simulink model "single_camera_xy_tracking_5dof"  (R2025b)
settings: Solver=FixedStepDiscrete  StartTime=0  StopTime=T_end  FixedStep=Ts  RelTol=1e-3
InitFcn:
  | % 获取顶层模型所在文件夹
  | root_model_file = get_param(bdroot,'FileName');
  | root_folder = fileparts(root_model_file);
  | % 定位config目录：模型目录上跳一层 → simulink → config
  | func_folder = fullfile(root_folder,'..','config');
  | addpath(func_folder);
  | % 拼接初始化脚本完整路径
  | init_script = fullfile(func_folder,'init_single_camera_xy_tracking_5dof.m');
  | run(init_script);
values from neighbouring files (symbols this model uses):
  Kpx = parameters(3)    [build_single_camera_joint_velocity_direct.m]    (also in build_single_camera_joint_velocity_direct1.m)
  Kpy = parameters(4);",  "k_ff=parameters(5)    [build_single_camera_joint_velocity_direct.m]    (also in build_single_camera_joint_velocity_direct1.m)
  Z_hat = parameters(2)    [build_single_camera_joint_velocity_direct.m]    (also in build_single_camera_joint_velocity_direct1.m)
undefined symbols (not defined in the file or in its folder): a_xy_max, adapt_max, camera_velocity_feedback_timeout_sec, controller_enable, cx, cy, data, data_SL_Info, ekf_gate_threshold, ekf_reset_timeout_sec, enable_adaptation, enable_ekf_feedforward, enable_proportional, fx, fy, gamma_adapt, joint_state_timeout_sec, k_ff, P0, Q_ekf, R_ekf, sigma_adapt, target_timeout_sec, Ts, v_xy_max
libraries: ros2lib x4, robotmaniplib x2
Description:
  | 5-DOF camera EKF/controller: vx, vy, wx, wy, wz enabled; vz=0.
settings Model: Creator=ASUS  LastModifiedBy=harry
settings DataIOCC: SignalLogging=off

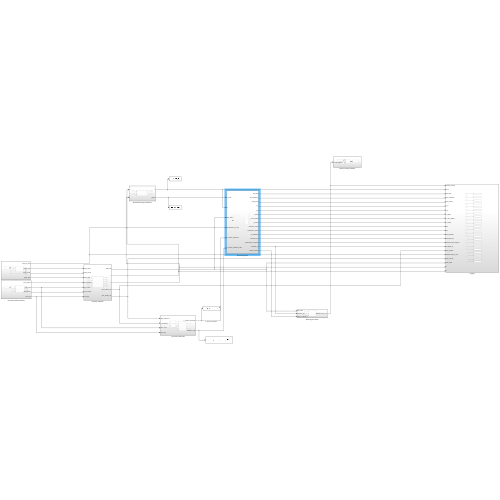
[thumbnail: Simulink's stored preview of the top-level diagram]
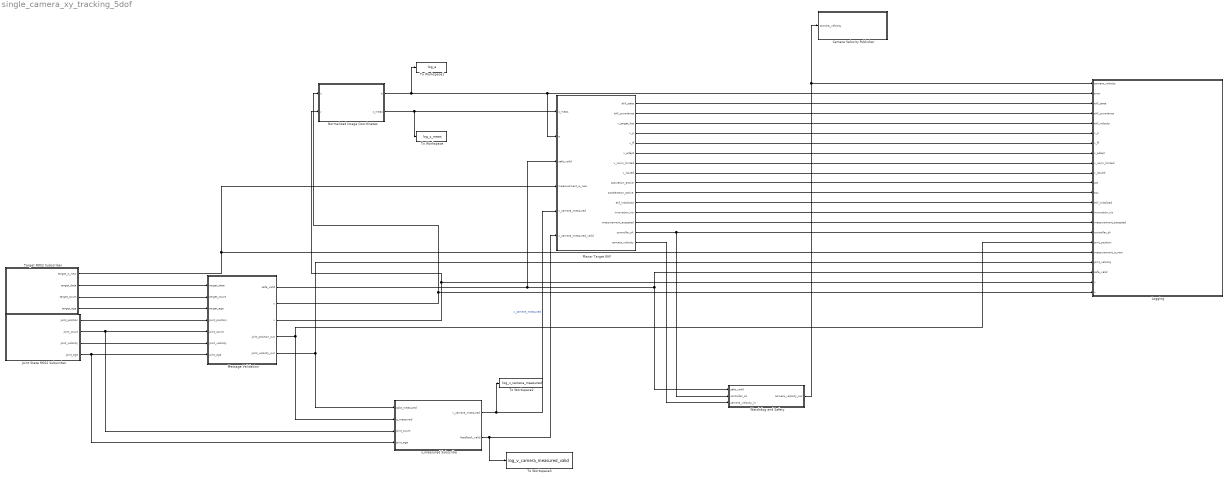
== system single_camera_xy_tracking_5dof ==
  Camera Velocity Publisher : Subsystem
  Joint State ROS2 Subscriber : Subsystem
  Logging : Subsystem
  Message Validation : Subsystem
  Normalized Image Coordinates : Subsystem
  Planar Target EKF : Subsystem
  Target ROS2 Subscriber : Subsystem
  To Workspace : ToWorkspace  VariableName=log_z_meas  SaveFormat=Timeseries  SampleTime=-1
  To Workspace1 : ToWorkspace  VariableName=log_e  SaveFormat=Timeseries  SampleTime=-1
  To Workspace2 : ToWorkspace  VariableName=log_v_camera_measured  SaveFormat=Timeseries  SampleTime=-1
  To Workspace3 : ToWorkspace  VariableName=log_v_camera_measured_valid  SaveFormat=Timeseries  SampleTime=-1
  Watchdog and Safety : Subsystem
  v_measured Subscribe : Subsystem
  wires:
  Target ROS2 Subscriber/4(target_age) -> Message Validation/3(target_age)
  Target ROS2 Subscriber/2(target_data) -> Message Validation/1(target_data)
  Target ROS2 Subscriber/3(target_count) -> Message Validation/2(target_count)
  Planar Target EKF/3(v_target_hat) -> Logging/5(ekf_velocity)
  Message Validation/2(u) -> Normalized Image Coordinates/1(u), Logging/22(u)
  Planar Target EKF/14(controller_ok) -> Watchdog and Safety/2(controller_ok), Logging/16(controller_ok)
  Planar Target EKF/6(v_adapt) -> Logging/8(v_adapt)
  Joint State ROS2 Subscriber/4(joint_age) -> v_measured Subscribe/4(joint_age), Message Validation/7(joint_age)
  Joint State ROS2 Subscriber/2(joint_count) -> v_measured Subscribe/3(joint_count), Message Validation/5(joint_count)
  Joint State ROS2 Subscriber/1(joint_position) -> Message Validation/4(joint_position)
  Joint State ROS2 Subscriber/3(joint_velocity) -> Message Validation/6(joint_velocity)
  Message Validation/1(safe_valid) -> Logging/20(safe_valid), Watchdog and Safety/1(safe_valid), Planar Target EKF/3(safe_valid)
  Message Validation/3(v) -> Normalized Image Coordinates/2(v), Logging/21(v)
  Message Validation/4(joint_position_out) -> v_measured Subscribe/2(q_measured), Logging/17(joint_position)
  Message Validation/5(joint_velocity_out) -> v_measured Subscribe/1(qdot_measured), Logging/19(joint_velocity)
  Normalized Image Coordinates/1(e) -> To Workspace1/1, Logging/2(error), Planar Target EKF/2(e)
  Normalized Image Coordinates/2(z_meas) -> To Workspace/1, Planar Target EKF/1(z_meas)
  Planar Target EKF/1(ekf_state) -> Logging/3(ekf_state)
  Planar Target EKF/2(ekf_covariance) -> Logging/4(ekf_covariance)
  Planar Target EKF/13(measurement_accepted) -> Logging/15(measurement_accepted)
  Planar Target EKF/9(saturation_active) -> Logging/11(sat)
  Planar Target EKF/10(acceleration_active) -> Logging/12(acc)
  Planar Target EKF/11(ekf_initialized) -> Logging/13(ekf_initialized)
  Planar Target EKF/12(innovation_nis) -> Logging/14(innovation_nis)
  Planar Target EKF/4(v_p) -> Logging/6(v_p)
  Planar Target EKF/5(v_ff) -> Logging/7(v_ff)
  Planar Target EKF/8(v_issued) -> Logging/10(v_issued)
  Planar Target EKF/15(camera_velocity) -> Watchdog and Safety/3(camera_velocity_in)
  Watchdog and Safety/1(camera_velocity_out) -> Camera Velocity Publisher/1(camera_velocity), Logging/1(camera_velocity)
  Target ROS2 Subscriber/1(target_is_new) -> Planar Target EKF/4(measurement_is_new), Logging/18(measurement_is_new)
  v_measured Subscribe/1(v_camera_measured) -> To Workspace2/1, Planar Target EKF/5(v_camera_measured)  "v_camera_measured"
  v_measured Subscribe/2(feedback_valid) -> To Workspace3/1, Planar Target EKF/6(v_camera_measured_valid)
  Planar Target EKF/7(v_norm_limited) -> Logging/9(v_norm_limited)

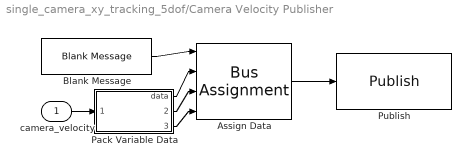
== system single_camera_xy_tracking_5dof/Camera Velocity Publisher ==
  camera_velocity : Inport
  Assign Data : BusAssignment  AssignedSignals=data,data_SL_Info.CurrentLength,data_SL_Info.ReceivedLength
  Blank Message : ros2lib/Blank Message  messageClass=Message  entityType=std_msgs/Float64MultiArray  messageType=std_msgs/Float64MultiArray  SampleTime=Ts
  Pack Variable Data : MATLAB Function  TreatAsAtomicUnit=on
  Publish : ros2lib/Publish  topicSource=Select from ROS network  topic=/simulink/camera_velocity  messageType=std_msgs/Float64MultiArray  QOSHistory=Keep last  QOSDepth=1  QOSReliability=Reliable  QOSDurability=Volatile  QOSDeadline=Inf  QOSLifespan=Inf  QOSLiveliness=Automatic  QOSLeaseDuration=Inf  QOSAvoidROSNamespaceConventions=off
  wires:
  Blank Message/1 -> Assign Data/1
  Assign Data/1 -> Publish/1
  camera_velocity/1 -> Pack Variable Data/1(camera_velocity)
  Pack Variable Data/1(data) -> Assign Data/2
  Pack Variable Data/2(current_length) -> Assign Data/3
  Pack Variable Data/3(received_length) -> Assign Data/4

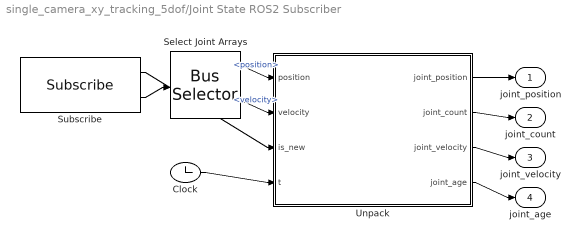
== system single_camera_xy_tracking_5dof/Joint State ROS2 Subscriber ==
  Clock : Clock
  Select Joint Arrays : BusSelector  OutputSignals=position,velocity
  Subscribe : ros2lib/Subscribe  topicSource=Select from ROS network  topic=/franka/joint_states  messageType=sensor_msgs/JointState  sampleTime=Ts  QOSHistory=Keep last  QOSDepth=1  QOSReliability=Best effort  QOSDurability=Volatile  QOSDeadline=Inf  QOSLifespan=Inf  QOSLiveliness=Automatic  QOSLeaseDuration=Inf  QOSAvoidROSNamespaceConventions=off
  Unpack : MATLAB Function  TreatAsAtomicUnit=on
  joint_position : Outport
  joint_count : Outport  Port=2
  joint_velocity : Outport  Port=3
  joint_age : Outport  Port=4
  wires:
  Unpack/1(joint_position) -> joint_position/1
  Unpack/2(joint_count) -> joint_count/1
  Unpack/3(joint_velocity) -> joint_velocity/1
  Unpack/4(joint_age) -> joint_age/1
  Select Joint Arrays/1 -> Unpack/1(position)  "<position>"
  Select Joint Arrays/2 -> Unpack/2(velocity)  "<velocity>"
  Clock/1 -> Unpack/4(t)
  Subscribe/2 -> Select Joint Arrays/1
  Subscribe/1 -> Unpack/3(is_new)

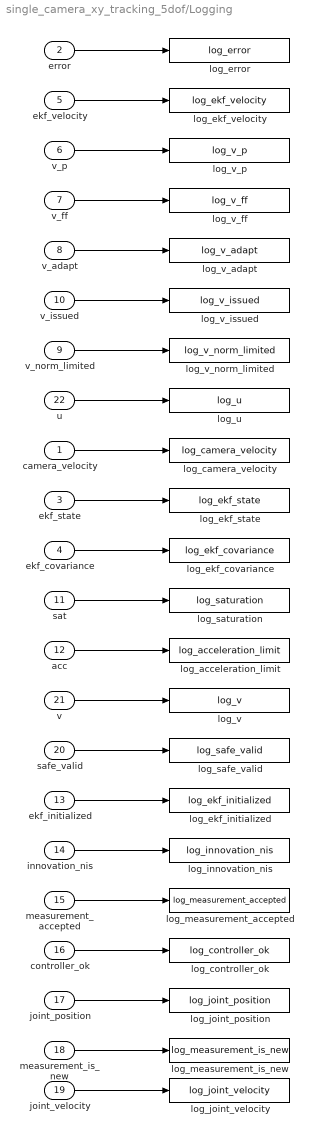
== system single_camera_xy_tracking_5dof/Logging ==
  camera_velocity : Inport
  error : Inport  Port=2
  ekf_state : Inport  Port=3
  ekf_covariance : Inport  Port=4
  ekf_velocity : Inport  Port=5
  v_p : Inport  Port=6
  v_ff : Inport  Port=7
  v_adapt : Inport  Port=8
  v_norm_limited : Inport  Port=9
  v_issued : Inport  Port=10
  sat : Inport  Port=11
  acc : Inport  Port=12
  ekf_initialized : Inport  Port=13
  innovation_nis : Inport  Port=14
  measurement_accepted : Inport  Port=15
  controller_ok : Inport  Port=16
  joint_position : Inport  Port=17
  measurement_is_new : Inport  Port=18
  joint_velocity : Inport  Port=19
  safe_valid : Inport  Port=20
  v : Inport  Port=21
  u : Inport  Port=22
  log_acceleration_limit : ToWorkspace  VariableName=log_acceleration_limit  SaveFormat=Structure With Time  SampleTime=-1
  log_camera_velocity : ToWorkspace  VariableName=log_camera_velocity  SaveFormat=Structure With Time  SampleTime=-1
  log_controller_ok : ToWorkspace  VariableName=log_controller_ok  SaveFormat=Structure With Time  SampleTime=-1
  log_ekf_covariance : ToWorkspace  VariableName=log_ekf_covariance  SaveFormat=Structure With Time  SampleTime=-1
  log_ekf_initialized : ToWorkspace  VariableName=log_ekf_initialized  SaveFormat=Structure With Time  SampleTime=-1
  log_ekf_state : ToWorkspace  VariableName=log_ekf_state  SaveFormat=Structure With Time  SampleTime=-1
  log_ekf_velocity : ToWorkspace  VariableName=log_ekf_velocity  SaveFormat=Structure With Time  SampleTime=-1
  log_error : ToWorkspace  VariableName=log_error  SaveFormat=Structure With Time  SampleTime=-1
  log_innovation_nis : ToWorkspace  VariableName=log_innovation_nis  SaveFormat=Structure With Time  SampleTime=-1
  log_joint_position : ToWorkspace  VariableName=log_joint_position  SaveFormat=Structure With Time  SampleTime=-1
  log_joint_velocity : ToWorkspace  VariableName=log_joint_velocity  SaveFormat=Structure With Time  SampleTime=-1
  log_measurement_accepted : ToWorkspace  VariableName=log_measurement_accepted  SaveFormat=Structure With Time  SampleTime=-1
  log_measurement_is_new : ToWorkspace  VariableName=log_measurement_is_new  SaveFormat=Structure With Time  SampleTime=-1
  log_safe_valid : ToWorkspace  VariableName=log_safe_valid  SaveFormat=Structure With Time  SampleTime=-1
  log_saturation : ToWorkspace  VariableName=log_saturation  SaveFormat=Structure With Time  SampleTime=-1
  log_u : ToWorkspace  VariableName=log_u  SaveFormat=Structure With Time  SampleTime=-1
  log_v : ToWorkspace  VariableName=log_v  SaveFormat=Structure With Time  SampleTime=-1
  log_v_adapt : ToWorkspace  VariableName=log_v_adapt  SaveFormat=Structure With Time  SampleTime=-1
  log_v_ff : ToWorkspace  VariableName=log_v_ff  SaveFormat=Structure With Time  SampleTime=-1
  log_v_issued : ToWorkspace  VariableName=log_v_issued  SaveFormat=Structure With Time  SampleTime=-1
  log_v_norm_limited : ToWorkspace  VariableName=log_v_norm_limited  SaveFormat=Structure With Time  SampleTime=-1
  log_v_p : ToWorkspace  VariableName=log_v_p  SaveFormat=Structure With Time  SampleTime=-1
  wires:
  error/1 -> log_error/1
  ekf_velocity/1 -> log_ekf_velocity/1
  v_p/1 -> log_v_p/1
  v_ff/1 -> log_v_ff/1
  v_adapt/1 -> log_v_adapt/1
  v_issued/1 -> log_v_issued/1
  u/1 -> log_u/1
  camera_velocity/1 -> log_camera_velocity/1
  ekf_state/1 -> log_ekf_state/1
  ekf_covariance/1 -> log_ekf_covariance/1
  sat/1 -> log_saturation/1
  acc/1 -> log_acceleration_limit/1
  v/1 -> log_v/1
  safe_valid/1 -> log_safe_valid/1
  ekf_initialized/1 -> log_ekf_initialized/1
  innovation_nis/1 -> log_innovation_nis/1
  measurement_accepted/1 -> log_measurement_accepted/1
  controller_ok/1 -> log_controller_ok/1
  joint_position/1 -> log_joint_position/1
  joint_velocity/1 -> log_joint_velocity/1
  measurement_is_new/1 -> log_measurement_is_new/1
  v_norm_limited/1 -> log_v_norm_limited/1

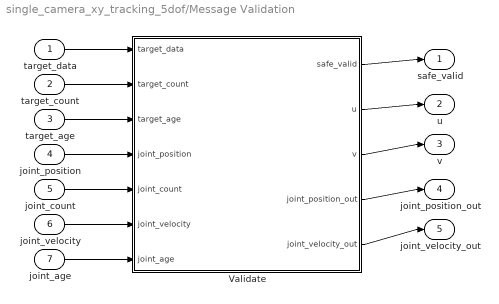
== system single_camera_xy_tracking_5dof/Message Validation ==
  target_data : Inport
  target_count : Inport  Port=2
  target_age : Inport  Port=3
  joint_position : Inport  Port=4
  joint_count : Inport  Port=5
  joint_velocity : Inport  Port=6
  joint_age : Inport  Port=7
  Validate : MATLAB Function  TreatAsAtomicUnit=on
  safe_valid : Outport
  u : Outport  Port=2
  v : Outport  Port=3
  joint_position_out : Outport  Port=4
  joint_velocity_out : Outport  Port=5
  wires:
  Validate/1(safe_valid) -> safe_valid/1
  Validate/2(u) -> u/1
  Validate/3(v) -> v/1
  Validate/4(joint_position_out) -> joint_position_out/1
  Validate/5(joint_velocity_out) -> joint_velocity_out/1
  target_data/1 -> Validate/1(target_data)
  target_count/1 -> Validate/2(target_count)
  target_age/1 -> Validate/3(target_age)
  joint_position/1 -> Validate/4(joint_position)
  joint_count/1 -> Validate/5(joint_count)
  joint_velocity/1 -> Validate/6(joint_velocity)
  joint_age/1 -> Validate/7(joint_age)

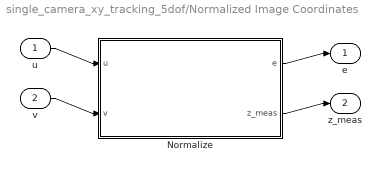
== system single_camera_xy_tracking_5dof/Normalized Image Coordinates ==
  u : Inport
  v : Inport  Port=2
  Normalize : MATLAB Function  TreatAsAtomicUnit=on
  e : Outport
  z_meas : Outport  Port=2
  wires:
  u/1 -> Normalize/1(u)
  v/1 -> Normalize/2(v)
  Normalize/1(e) -> e/1
  Normalize/2(z_meas) -> z_meas/1

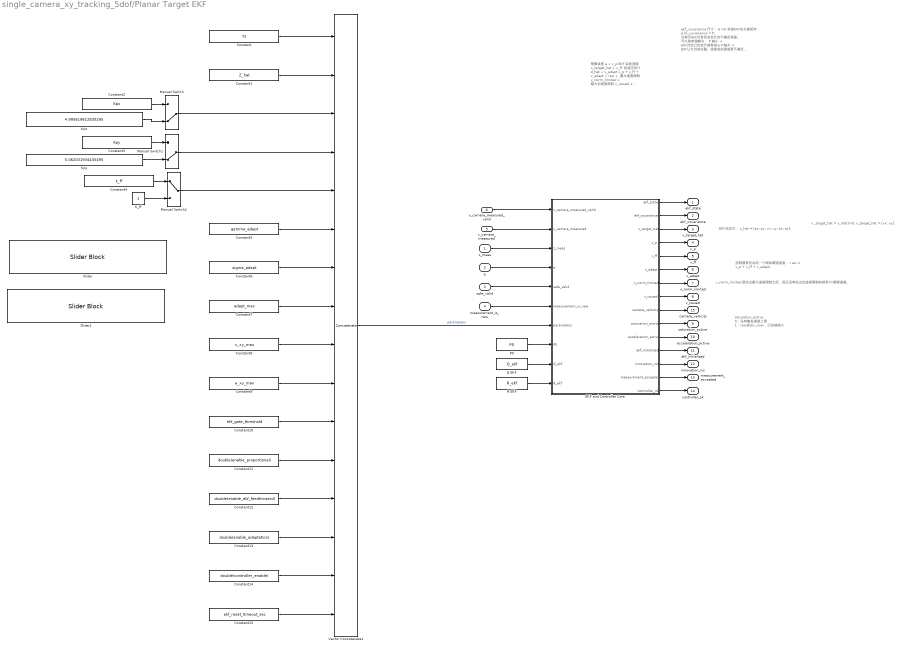
== system single_camera_xy_tracking_5dof/Planar Target EKF ==
  note: saturation_active
      | 0：没有触发速度上限
      | 1：raw超过v_max，已经被缩小
  note: ekf_covariance
      | 尺寸：
      | 6 ×6
      | 就是EKF协方差矩阵：
      | e kf_covariance = P;
      | 它表示EKF对各状态估计的不确定程度。
      | 可以简单理解为：
      | P 越小
      | → EKF对自己的估计越有信心
      |
      | P越大
      | → EKF认为当前位置、速度或加速度更不确定
      | 重点可以观察：
      | d iag(P)
      | 也就是：
      | 位 置方差
      | 速度方差
      | 加速度方差
  note: 图像误差 e
      |     ↓
      | v_p
      |
      | EKF目标速度 v_target_hat
      |     ↓
      | v_ff
      |
      | 自适应估计 d_hat
      |     ↓
      | v_adapt
      |
      | v_p + v_ff + v_adapt
      |     ↓
      | raw
      |     ↓ 最大速度限制
      | v_norm_limited
      |     ↓ 最大加速度限制
      | v_issued
      |     ↓ 扩展为6维
      | camera_velocity
  note: EKF状态为： x_hat = [px; py; vx; vy; ax; ay];
  note: v _target_hat = x_hat(3:4); v_target_hat = [vx; vy];
  note: 控制器首先合成一个原始期望速度：
      | r aw = v_p + v_ff + v_adapt;
  note: v_norm_limited 是经过最大速度限制之后、但还没有经过加速度限制的相机XY期望速度。
  z_meas : Inport
  e : Inport  Port=2
  safe_valid : Inport  Port=3
  measurement_is_new : Inport  Port=4
  v_camera_measured : Inport  Port=5
  v_camera_measured_valid : Inport  Port=6
  Constant : Constant  Value=Ts
  Constant1 : Constant  Value=Z_hat
  Constant10 : Constant  Value=ekf_gate_threshold
  Constant11 : Constant  Value=double(enable_proportional)
  Constant12 : Constant  Value=double(enable_ekf_feedforward)
  Constant13 : Constant  Value=double(enable_adaptation)
  Constant14 : Constant  Value=double(controller_enable)
  Constant15 : Constant  Value=ekf_reset_timeout_sec
  Constant2 : Constant  Value=Kpx
  Constant3 : Constant  Value=Kpy
  Constant4 : Constant  Value=k_ff
  Constant5 : Constant  Value=gamma_adapt
  Constant6 : Constant  Value=sigma_adapt
  Constant7 : Constant  Value=adapt_max
  Constant8 : Constant  Value=v_xy_max
  Constant9 : Constant  Value=a_xy_max
  EKF and Controller Core : MATLAB Function  TreatAsAtomicUnit=on
  K_ff : Constant
  Kpx : Constant  Value=4.995619612830295
  Kpy : Constant  Value=5.062031934435495
  Manual Switch : ManualSwitch  CurrentSetting=0
  Manual Switch1 : ManualSwitch  CurrentSetting=0
  Manual Switch2 : ManualSwitch
  P0 : Constant  Value=P0
  Q EKF : Constant  Value=Q_ekf
  R EKF : Constant  Value=R_ekf
  Slider : SliderBlock  ScaleMax=10
  Slider1 : SliderBlock  ScaleMax=10
  Vector Concatenate1 : Concatenate  NumInputs=16
  ekf_state : Outport
  ekf_covariance : Outport  Port=2
  v_target_hat : Outport  Port=3
  v_p : Outport  Port=4
  v_ff : Outport  Port=5
  v_adapt : Outport  Port=6
  v_norm_limited : Outport  Port=7
  v_issued : Outport  Port=8
  saturation_active : Outport  Port=9
  acceleration_active : Outport  Port=10
  ekf_initialized : Outport  Port=11
  innovation_nis : Outport  Port=12
  measurement_accepted : Outport  Port=13
  controller_ok : Outport  Port=14
  camera_velocity : Outport  Port=15
  wires:
  EKF and Controller Core/1(ekf_state) -> ekf_state/1
  EKF and Controller Core/2(ekf_covariance) -> ekf_covariance/1
  EKF and Controller Core/3(v_target_hat) -> v_target_hat/1
  EKF and Controller Core/4(v_p) -> v_p/1
  EKF and Controller Core/5(v_ff) -> v_ff/1
  EKF and Controller Core/6(v_adapt) -> v_adapt/1
  EKF and Controller Core/7(v_norm_limited) -> v_norm_limited/1
  EKF and Controller Core/8(v_issued) -> v_issued/1
  EKF and Controller Core/9(camera_velocity) -> camera_velocity/1
  EKF and Controller Core/10(saturation_active) -> saturation_active/1
  EKF and Controller Core/11(acceleration_active) -> acceleration_active/1
  EKF and Controller Core/12(ekf_initialized) -> ekf_initialized/1
  EKF and Controller Core/13(innovation_nis) -> innovation_nis/1
  EKF and Controller Core/14(measurement_accepted) -> measurement_accepted/1
  EKF and Controller Core/15(controller_ok) -> controller_ok/1
  z_meas/1 -> EKF and Controller Core/3(z_meas)
  e/1 -> EKF and Controller Core/4(e)
  safe_valid/1 -> EKF and Controller Core/5(safe_valid)
  measurement_is_new/1 -> EKF and Controller Core/6(measurement_is_new)
  Vector Concatenate1/1 -> EKF and Controller Core/7(parameters)  "parameters"
  P0/1 -> EKF and Controller Core/8(P0)
  Q EKF/1 -> EKF and Controller Core/9(Q_ekf)
  R EKF/1 -> EKF and Controller Core/10(R_ekf)
  Constant/1 -> Vector Concatenate1/1
  Constant1/1 -> Vector Concatenate1/2
  Constant5/1 -> Vector Concatenate1/6
  Constant6/1 -> Vector Concatenate1/7
  Constant7/1 -> Vector Concatenate1/8
  Constant8/1 -> Vector Concatenate1/9
  Constant9/1 -> Vector Concatenate1/10
  Constant10/1 -> Vector Concatenate1/11
  Constant11/1 -> Vector Concatenate1/12
  Constant12/1 -> Vector Concatenate1/13
  Constant13/1 -> Vector Concatenate1/14
  Constant14/1 -> Vector Concatenate1/15
  Constant15/1 -> Vector Concatenate1/16
  v_camera_measured/1 -> EKF and Controller Core/2(v_camera_measured)
  v_camera_measured_valid/1 -> EKF and Controller Core/1(v_camera_measured_valid)
  Constant2/1 -> Manual Switch/1
  Manual Switch/1 -> Vector Concatenate1/3
  Kpx/1 -> Manual Switch/2
  Kpy/1 -> Manual Switch1/2
  Constant3/1 -> Manual Switch1/1
  Manual Switch1/1 -> Vector Concatenate1/4
  Constant4/1 -> Manual Switch2/1
  Manual Switch2/1 -> Vector Concatenate1/5
  K_ff/1 -> Manual Switch2/2

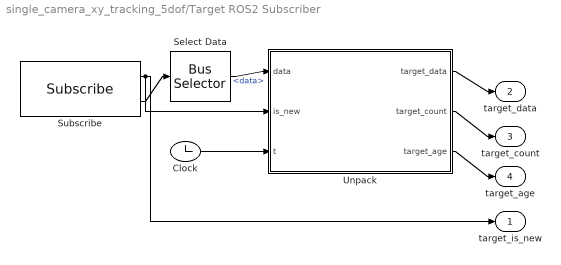
== system single_camera_xy_tracking_5dof/Target ROS2 Subscriber ==
  Clock : Clock
  Select Data : BusSelector  OutputSignals=data
  Subscribe : ros2lib/Subscribe  topicSource=Select from ROS network  topic=/apriltag_detector/target_position  messageType=std_msgs/Float64MultiArray  sampleTime=Ts  QOSHistory=Keep last  QOSDepth=1  QOSReliability=Best effort  QOSDurability=Volatile  QOSDeadline=Inf  QOSLifespan=Inf  QOSLiveliness=Automatic  QOSLeaseDuration=Inf  QOSAvoidROSNamespaceConventions=off
  Unpack : MATLAB Function  TreatAsAtomicUnit=on
  target_is_new : Outport
  target_data : Outport  Port=2
  target_count : Outport  Port=3
  target_age : Outport  Port=4
  wires:
  Unpack/1(target_data) -> target_data/1
  Unpack/2(target_count) -> target_count/1
  Unpack/3(target_age) -> target_age/1
  Select Data/1 -> Unpack/1(data)  "<data>"
  Clock/1 -> Unpack/3(t)
  Subscribe/2 -> Select Data/1
  Subscribe/1 -> Unpack/2(is_new), target_is_new/1

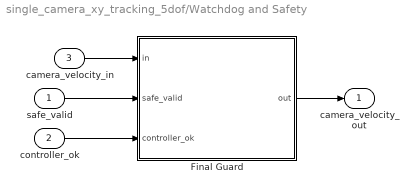
== system single_camera_xy_tracking_5dof/Watchdog and Safety ==
  safe_valid : Inport
  controller_ok : Inport  Port=2
  camera_velocity_in : Inport  Port=3
  Final Guard : MATLAB Function  TreatAsAtomicUnit=on
  camera_velocity_out : Outport
  wires:
  camera_velocity_in/1 -> Final Guard/1(in)
  safe_valid/1 -> Final Guard/2(safe_valid)
  controller_ok/1 -> Final Guard/3(controller_ok)
  Final Guard/1(out) -> camera_velocity_out/1

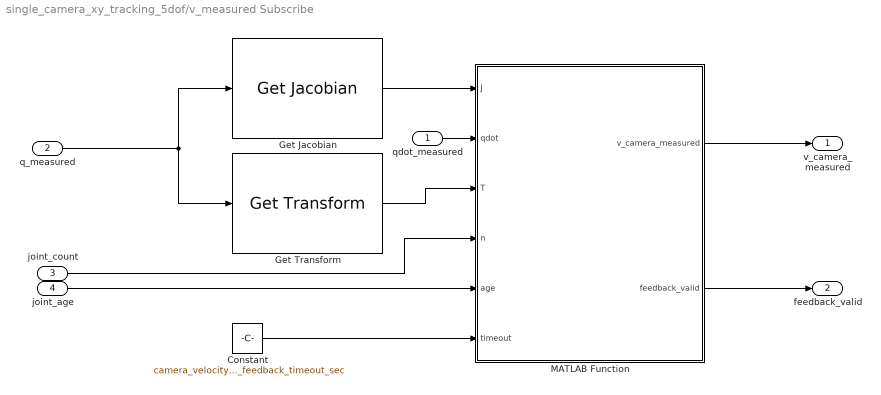
== system single_camera_xy_tracking_5dof/v_measured Subscribe ==
  qdot_measured : Inport
  q_measured : Inport  Port=2
  joint_count : Inport  Port=3
  joint_age : Inport  Port=4
  Constant : Constant  Value=camera_velocity_feedback_timeout_sec
  Get Jacobian : robotmaniplib/Get Jacobian  RigidBodyTree=fr3_camera_robot  EndEffector=camera_link  SimulateUsing=Interpreted execution
  Get Transform : robotmaniplib/Get Transform  RigidBodyTree=fr3_camera_robot  SourceBody=camera_link  TargetBody=base  SimulateUsing=Interpreted execution
  MATLAB Function : MATLAB Function  TreatAsAtomicUnit=on
  v_camera_measured : Outport
  feedback_valid : Outport  Port=2
  wires:
  q_measured/1 -> Get Transform/1, Get Jacobian/1
  qdot_measured/1 -> MATLAB Function/2(qdot)
  Get Jacobian/1 -> MATLAB Function/1(J)
  Get Transform/1 -> MATLAB Function/3(T)
  joint_count/1 -> MATLAB Function/4(n)
  joint_age/1 -> MATLAB Function/5(age)
  Constant/1 -> MATLAB Function/6(timeout)
  MATLAB Function/1(v_camera_measured) -> v_camera_measured/1
  MATLAB Function/2(feedback_valid) -> feedback_valid/1

== matlab function single_camera_xy_tracking_5dof/Planar Target EKF/EKF and Controller Core ==
  data: v_camera_measured_valid input; v_camera_measured input size=[5 1]; z_meas input size=[2 1]; ekf_state output size=[6 1]; e input size=[2 1]; safe_valid input size=1; measurement_is_new input; parameters input size=[16 1]; P0 input size=[6 6]; Q_ekf input size=[6 6]; R_ekf input size=[2 2]; ekf_covariance output size=[6 6]; v_target_hat output size=[2 1]; v_p output size=[2 1]; v_ff output size=[2 1]; v_adapt output size=[2 1]; v_norm_limited output size=[2 1]; v_issued output size=[2 1]; camera_velocity output size=[6 1]; saturation_active output size=1; acceleration_active output size=1; ekf_initialized output size=1; innovation_nis output size=1; measurement_accepted output size=1; controller_ok output size=1
function [ekf_state,ekf_covariance,v_target_hat,v_p,v_ff,v_adapt, ...
    v_norm_limited,v_issued,camera_velocity,saturation_active, ...
    acceleration_active,ekf_initialized,innovation_nis, ...
    measurement_accepted,controller_ok]=fcn( ...
    v_camera_measured_valid,v_camera_measured,z_meas,e,safe_valid, ...
    measurement_is_new,parameters,P0,Q_ekf,R_ekf)
%#codegen
% EKF=[X Y Vx Vy Ax Ay]'；相机反馈=[vx vy wx wy wz]'，仅 vz=0。
persistent x P d v_prev p_cam bad_time initialized e_hold
if isempty(initialized)
    x=zeros(6,1); P=P0; d=zeros(2,1); v_prev=zeros(2,1);
    p_cam=zeros(2,1); bad_time=0; initialized=false; e_hold=zeros(2,1);
end

Ts=parameters(1); Z=parameters(2); Kp=parameters(3:4);
kff=parameters(5); gamma=parameters(6); sigma=parameters(7);
dmax=parameters(8); vmax=parameters(9); amax=parameters(10);
gate=parameters(11); enP=parameters(12)>.5; enFF=parameters(13)>.5;
enA=parameters(14)>.5; enabled=parameters(15)>.5; timeout=parameters(16);
measurement_is_new=measurement_is_new>.5;

F=[1 0 Ts 0 Ts^2/2 0;0 1 0 Ts 0 Ts^2/2; ...
   0 0 1 0 Ts 0;0 0 0 1 0 Ts;0 0 0 0 1 0;0 0 0 0 0 1];
H=[eye(2) zeros(2,4)]; I=eye(6);

% 雅可比反馈在相机系下补偿图像平移与旋转。
twist_ok=v_camera_measured_valid>.5 && numel(v_camera_measured)==5 && ...
    all(isfinite(v_camera_measured(:)));
twist=[v_prev;0;0;0];
if twist_ok, twist=reshape(v_camera_measured,5,1); end
s=e_hold;
if numel(e)==2 && all(isfinite(e(:))), s=reshape(e,2,1); end
vx=twist(1); vy=twist(2); wx=twist(3); wy=twist(4); wz=twist(5);
p_cam=p_cam+Ts*[vx-Z*s(1)*s(2)*wx+Z*(1+s(1)^2)*wy-Z*s(2)*wz; ...
    vy-Z*(1+s(2)^2)*wx+Z*s(1)*s(2)*wy+Z*s(1)*wz];
omega=zeros(3,1); if twist_ok, omega=twist(3:5); end

param_ok=all(isfinite(parameters(:))) && all(isfinite(P0(:))) && ...
    all(isfinite(Q_ekf(:))) && all(isfinite(R_ekf(:))) && ...
    Ts>0 && Z>0 && vmax>0 && amax>0 && timeout>=Ts;
input_ok=safe_valid && enabled && param_ok && ...
    all(isfinite(z_meas(:))) && all(isfinite(e(:)));

% 默认输出。
ekf_state=x; ekf_covariance=P; v_target_hat=zeros(2,1);
v_p=zeros(2,1); v_ff=zeros(2,1); v_adapt=zeros(2,1);
v_norm_limited=zeros(2,1); v_issued=zeros(2,1);
camera_velocity=zeros(6,1); saturation_active=false;
acceleration_active=false; ekf_initialized=initialized;
innovation_nis=NaN; measurement_accepted=false; controller_ok=false;

if ~input_ok
    if initialized, x=F*x; P=F*P*F'+Q_ekf; P=(P+P')/2; end
    bad_time=bad_time+Ts; d(:)=0; v_prev(:)=0; e_hold(:)=0;
    state_ok=all(isfinite(x)) && all(isfinite(P(:))) && all(diag(P)>=0);
    if bad_time>=timeout || ~state_ok
        x(:)=0; P=P0; p_cam(:)=0; initialized=false;
    end
    ekf_state=x; ekf_covariance=P; v_target_hat=x(3:4);
    ekf_initialized=initialized; return
end
bad_time=0;

if ~initialized
    if ~measurement_is_new, return; end
    z=z_meas+p_cam; x=[z;zeros(4,1)]; P=P0;
    initialized=true; measurement_accepted=true; e_hold=e;
else
    xp=F*x; Pp=F*P*F'+Q_ekf; Pp=(Pp+Pp')/2; x=xp; P=Pp;
    if measurement_is_new
        e_hold=e; innovation=z_meas+p_cam-H*xp; S=H*Pp*H'+R_ekf;
        if all(isfinite(S(:))) && rcond(S)>1e-12
            innovation_nis=innovation'*(S\innovation);
        else
            innovation_nis=inf;
        end
        if isfinite(innovation_nis) && innovation_nis<=gate
            Kg=(Pp*H')/S; x=xp+Kg*innovation; A=I-Kg*H;
            P=A*Pp*A'+Kg*R_ekf*Kg'; P=(P+P')/2;
            measurement_accepted=true;
        end
    end
end

state_ok=all(isfinite(x)) && all(isfinite(P(:))) && ...
    all(diag(P)>=0) && norm(P-P','fro')<1e-6;
if ~state_ok
    x(:)=0; P=P0; d(:)=0; v_prev(:)=0; p_cam(:)=0;
    e_hold(:)=0; initialized=false; ekf_state=x;
    ekf_covariance=P; ekf_initialized=false; return
end

ekf_state=x; ekf_covariance=P; v_target_hat=x(3:4);
ekf_initialized=initialized;
if enP, v_p=Z*Kp.*e_hold; end
if enFF, v_ff=kff*v_target_hat; end
if enA
    d=max(0,1-sigma*Ts)*d+gamma*Z*e_hold*Ts;
    d=min(max(d,-dmax),dmax);
else
    d(:)=0;
end
v_adapt=d; raw=v_p+v_ff+v_adapt; nr=norm(raw);
saturation_active=nr>vmax;
if saturation_active, v_norm_limited=raw*(vmax/nr); else, v_norm_limited=raw; end
dv=v_norm_limited-v_prev; nd=norm(dv); step=amax*Ts;
acceleration_active=nd>step;
if acceleration_active, v_issued=v_prev+dv*(step/nd); else, v_issued=v_norm_limited; end

controller_ok=all(isfinite([v_p;v_ff;v_adapt;v_issued;omega]));
if controller_ok
    v_prev=v_issued;
    camera_velocity=[v_issued;0;omega]; % [vx vy 0 wx wy wz]'
else
    x(:)=0; P=P0; d(:)=0; v_prev(:)=0; p_cam(:)=0; e_hold(:)=0;
    initialized=false; ekf_state=x; ekf_covariance=P;
    v_target_hat(:)=0; v_p(:)=0; v_ff(:)=0; v_adapt(:)=0;
    v_norm_limited(:)=0; v_issued(:)=0; camera_velocity(:)=0;
end
ekf_initialized=initialized;
end

== matlab function single_camera_xy_tracking_5dof/Watchdog and Safety/Final Guard ==
  data: in input size=[6 1]; out output size=[6 1]; safe_valid input size=1; controller_ok input size=1
function out=fcn(in,safe_valid,controller_ok)
%#codegen
out=zeros(6,1);
if safe_valid && controller_ok && all(isfinite(in))
    out=in; out(3)=0; % 仅禁止 vz，保留 vx、vy、wx、wy、wz
end
end

== matlab function single_camera_xy_tracking_5dof/Camera Velocity Publisher/Pack Variable Data ==
  data: camera_velocity input size=[6 1]; data output size=[128 1]; current_length output size=1; received_length output size=1
function [data,current_length,received_length] = fcn(camera_velocity)
%#codegen
data=zeros(128,1); data(1:6)=camera_velocity;
current_length=uint32(6); received_length=uint32(6);
end

== matlab function single_camera_xy_tracking_5dof/Target ROS2 Subscriber/Unpack ==
  data: data input; target_data output size=[3 1]; is_new input size=1; t input size=1; target_count output size=1; target_age output size=1
function [target_data,target_count,target_age] = fcn(data,is_new,t)
%#codegen
persistent last_data last_count last_time
if isempty(last_count), last_data=zeros(3,1); last_count=0.0; last_time=-1.0e6; end
if is_new
    n=numel(data); last_data=zeros(3,1);
    if n>=1, last_data(1)=data(1); end
    if n>=2, last_data(2)=data(2); end
    if n>=3, last_data(3)=data(3); end
    last_count=double(n); last_time=t;
end
target_data=last_data; target_count=last_count; target_age=max(0.0,t-last_time);
end

== matlab function single_camera_xy_tracking_5dof/v_measured Subscribe/MATLAB Function ==
  data: J input; v_camera_measured output size=[5 1]; qdot input; T input; n input; age input; timeout input; feedback_valid output
function [v_camera_measured,feedback_valid] = fcn(J,qdot,T,n,age,timeout)
%#codegen
% geometricJacobian: [wx wy wz vx vy vz]'，统一转到相机坐标系。
v_camera_measured=zeros(5,1); feedback_valid=false;
qdot=reshape(qdot,7,1);
if n<7 || ~isfinite(age) || age>timeout || any(~isfinite(qdot)) || ...
        any(~isfinite(J(:))) || any(~isfinite(T(:))) || ...
        ~isequal(size(J),[6 7]) || ~isequal(size(T),[4 4])
    return
end
twist=J*qdot; R=T(1:3,1:3);
w=R'*twist(1:3); v=R'*twist(4:6);
v_camera_measured=[v(1:2);w];
feedback_valid=all(isfinite(v_camera_measured));
if ~feedback_valid, v_camera_measured(:)=0; end
end

== matlab function single_camera_xy_tracking_5dof/Joint State ROS2 Subscriber/Unpack ==
  data: position input; joint_position output size=[7 1]; velocity input; is_new input size=1; t input size=1; joint_count output size=1; joint_velocity output size=[7 1]; joint_age output size=1
function [joint_position,joint_count,joint_velocity,joint_age] = fcn(position,velocity,is_new,t)
%#codegen
persistent last_q last_dq last_count last_time
if isempty(last_count), last_q=zeros(7,1); last_dq=zeros(7,1); last_count=0.0; last_time=-1.0e6; end
if is_new
    np=numel(position); nv=numel(velocity); last_q=zeros(7,1); last_dq=zeros(7,1);
    for k=1:min(np,7), last_q(k)=position(k); end
    for k=1:min(nv,7), last_dq(k)=velocity(k); end
    last_count=double(min(np,nv)); last_time=t;
end
joint_position=last_q; joint_count=last_count; joint_velocity=last_dq; joint_age=max(0.0,t-last_time);
end

== matlab function single_camera_xy_tracking_5dof/Message Validation/Validate ==
  data: target_data input size=[3 1]; safe_valid output size=1; target_count input size=1; target_age input size=1; joint_position input size=[7 1]; joint_count input size=1; joint_velocity input size=[7 1]; joint_age input size=1; u output size=1; v output size=1; joint_position_out output size=[7 1]; joint_velocity_out output size=[7 1]; target_timeout_sec parameter size=1; joint_state_timeout_sec parameter size=1
function [safe_valid,u,v,joint_position_out,joint_velocity_out] = fcn(target_data,target_count,target_age,joint_position,joint_count,joint_velocity,joint_age, target_timeout_sec, joint_state_timeout_sec)
%#codegen
u=0.0; v=0.0; joint_position_out=zeros(7,1); joint_velocity_out=zeros(7,1);
target_ok=target_count>=3 && target_data(1)>0.5 && isfinite(target_data(2)) && isfinite(target_data(3)) && isfinite(target_age) && target_age<=target_timeout_sec;
joint_ok=joint_count>=7 && all(isfinite(joint_position(:))) && all(isfinite(joint_velocity(:))) && isfinite(joint_age) && joint_age<=joint_state_timeout_sec;
if target_ok, u=target_data(2); v=target_data(3); end
if joint_ok, joint_position_out=joint_position; joint_velocity_out=joint_velocity; end
safe_valid=target_ok && joint_ok;
end

== matlab function single_camera_xy_tracking_5dof/Normalized Image Coordinates/Normalize ==
  data: u input size=1; e output size=[2 1]; v input size=1; z_meas output size=[2 1]; fx parameter size=1; fy parameter size=1; cx parameter size=1; cy parameter size=1; Z_hat parameter size=1
function [e,z_meas] = fcn(u,v, fx, fy, cx, cy, Z_hat)
%#codegen
ex=(u-cx)/fx; ey=(v-cy)/fy;
e=[ex;ey]; z_meas=Z_hat*e;
end
